simulink model "LPVmodel_wen0x2810x29"  (R2024a)
settings: Solver=VariableStepAuto  StartTime=0.0  StopTime=30  RelTol=1e-3
InitFcn:
  | run("gnrtLPVmodel.m")
StopFcn:
  | time = out.input.time;
  | u = out.input.data;      % N×1
  | y = out.output.data;     % N×5
  | allData = [time u y];
  | varNames = {'Time', 'w_f', 'F', 'N1', 'N2', 'P3', 'T5'};
  | T = array2table(allData, 'VariableNames', varNames);
  | writetable(T, 'fly_robot_LPV_data.csv');
values from neighbouring files (symbols this model uses):
  Actuator1 = c2d(Actuator1, Engine.SimConfig.Ts)    [gnrtLPVmodel.m]
  Engine =     [EngineData.mat]
  lpv_x0 = permute(Engine.PWLM.steadyState, [1 2 5 3 4])    [gnrtLPVmodel.m]
  schInd1 = 1    [gnrtLPVmodel.m]
undefined symbols (not defined in the file or in its folder): Plant_lpv
libraries: simulink x2, cstblocks x2
settings Model: Creator=LRC  LastModifiedBy=73626
settings SolverCC: AlgebraicLoopSolver=TrustRegion
settings DebuggingCC: UnconnectedInputMsg=warning  UnconnectedOutputMsg=warning  UnconnectedLineMsg=warning
settings ModelReferenceCC: EnableRefExpFcnMdlSchedulingChecks=on
settings SFSimCC: CustomCodeUndefinedFunction=UseInterfaceOnly
settings RTWCC: GPUComputeCapability=3.5

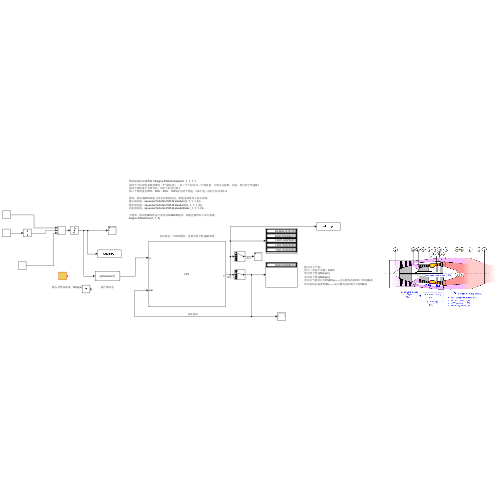
[thumbnail: Simulink's stored preview of the top-level diagram]
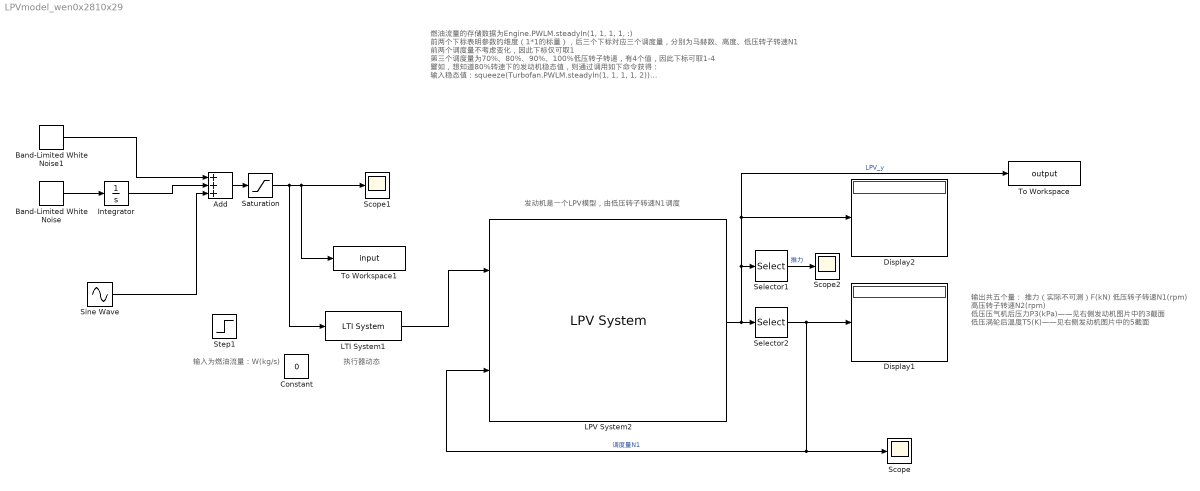
== system LPVmodel_wen0x2810x29 ==
  note: 燃油流量的存储数据为Engine.PWLM.steadyIn(1, 1, 1, 1, :)
      | 前两个下标表明参数的维度（1*1的标量），后三个下标对应三个调度量，分别为马赫数、高度、低压转子转速N1
      | 前两个调度量不考虑变化，因此下标仅可取1
      | 第三个调度量为70%、80%、90%、100%低压转子转速，有4个值，因此下标可取1-4
      |
      | 譬如，想知道80%转速下的发动机稳态值，则通过调用如下命令获得：
      | 输入稳态值：squeeze(Turbofan.PWLM.steadyIn(1, 1, 1, 1, 2))
      | 输出稳态值：squeeze(Turbofan.PWLM.steadyOut(:, 1, 1, 1, 2))
      | 状态稳态值：squeeze(Turbofan.PWLM.steadyState(:, 1, 1, 1, 2))
      |
      | 又譬如，想知道80%转速下的发动机ABCD矩阵，则通过调用如下命令获得：
      | Engine.PWLM.svm{1, 1, 2}
  note: 输出共五个量：
      | 推力（实际不可测）F(kN)
      | 低压转子转速N1(rpm)
      | 高压转子转速N2(rpm)
      | 低压压气机后压力P3(kPa)——见右侧发动机图片中的3截面
      | 低压涡轮后温度T5(K)——见右侧发动机图片中的5截面
  note: 输入为燃油流量：W(kg/s)
  note: 执行器动态
  note: 发动机是一个LPV模型，由低压转子转速N1调度
  Add : Sum  Inputs=+++
  Band-Limited White Noise : simulink/Sources/Band-Limited White Noise  Cov=[0.001]  Ts=0.1  seed=[23341]
  Band-Limited White Noise1 : simulink/Sources/Band-Limited White Noise  Cov=[0.01]  Ts=0.1  seed=[23341]
  Constant : Constant  Value=0
  Display1 : Display
  Display2 : Display
  Integrator : Integrator
  LPV System2 : cstblocks/Linear Parameter Varying/LPV System  sys=Plant_lpv  x0=lpv_x0(:, :, schInd1)  opSpecOption=Specify offsets as double arrays  uOffset=lpv_u0  yOffset=lpv_y0  xOffset=lpv_x0  opEquilOption=on  dxOffset=0  sysFixedOption=Custom value (specify below)  sysFixed=Plant_lpv(:, :, 1, 1)  AFixed=false  BFixed=false  CFixed=false  DFixed=false  uDelayFixed=true  yDelayFixed=true  iDelayFixed=true  IMethod=Linear  EMethod=Clip  IndexSearch=Binary search  IndexBegin=on  OutputX=off  OutputXdot=off  OutputLTI=off  OutputOP=off  DataType=double  InitBufferSize=1024  FixedBuffer=off  SimMode=Interpreted execution  Offset=struct
  LTI System1 : cstblocks/LTI System  sys=ss(Actuator1)  IC=[Engine.PWLM.steadyIn(1, :, 1, 1, schInd1)/ss(Actuator1).C]  PadeOrder=0
  Saturation : Saturate  UpperLimit=1.5827  LowerLimit=0.7
  Scope : Scope
  Scope1 : Scope
  Scope2 : Scope
  Selector1 : Selector  InputPortWidth=5  IndexOptions=Index vector (dialog)  Indices=1  OutputSizes=1
  Selector2 : Selector  InputPortWidth=5  IndexOptions=Index vector (dialog)  Indices=2  OutputSizes=1
  Sine Wave : Sin  Amplitude=0.7  Bias=0.7  SampleTime=0
  Step1 : Step  Before=Engine.PWLM.steadyIn(1, :, 1, 1, 1)  After=Engine.PWLM.steadyIn(1, :, 1, 1, end)  SampleTime=0
  To Workspace : ToWorkspace  VariableName=output  SaveFormat=Timeseries  SampleTime=0.001
  To Workspace1 : ToWorkspace  VariableName=input  SaveFormat=Timeseries  SampleTime=0.001
  wires:
  LTI System1/1 -> LPV System2/1
  Saturation/1 -> LTI System1/1, To Workspace1/1, Scope1/1
  LPV System2/1 -> To Workspace/1, Display2/1, Selector1/1, Selector2/1  "LPV_y"
  Selector2/1 -> Display1/1, Scope/1, LPV System2/2  "调度量N1"
  Band-Limited White Noise/1 -> Integrator/1
  Integrator/1 -> Add/2
  Band-Limited White Noise1/1 -> Add/1
  Sine Wave/1 -> Add/3
  Add/1 -> Saturation/1
  Selector1/1 -> Scope2/1  "推力"
